simulink library "UserBlocks"  (R2014a)
settings: Solver=ode45  SolverMode=SingleTasking  StartTime=0.0  StopTime=10.0  RelTol=1e-3
values from neighbouring files (symbols this model uses):
  a = param.a    [DSC_Control_Analysis.m]    (also in DSC_Control_Analysis_Exp.m; DSC_Speed_Control_Analysis.m; EmpiricalTireCurves.m = 1.35; FFW_Fx.m = sqrt(curvature/(2*clothoidLength)))
  b = 1.15    [EmpiricalTireCurves.m]
  Cfls = Cfl    [EC_params_nissan.m]
  Crls = Crl    [EC_params_nissan.m]
  d0 = CSTR.d0    [Ext_MPCPara.m]
  freq = Fs/2*linspace(0,1,NFFT/2)    [AACplottingcode.m]    (also in If_alpha_tp_observer.m; If_alpha_tp_observer_for_c_code.m; If_alpha_tp_observer_shoreline.m)
  Iz = param.Iz    [DSC_Control_Analysis.m]    (also in DSC_Control_Analysis_Exp.m; DSC_Speed_Control_Analysis.m; EmpiricalTireCurves.m = 1300)
  K = 10    [EC_params_nissan.m]
  Ks = -10    [EC_params_nissan.m]
  Ksl = -10    [EC_params_nissan.m]
  Kt = 40000    [EC_params_nissan.m]
  Ku = -40000    [EC_params_nissan.m]
  m = 1724    [EmpiricalTireCurves.m]
  mu_s = mu_p    (= 0.6)    [EC_params_nissan.m]    (also in EmpiricalTireCurves.m = 0.55)
  Ns = 10    [EC_params_nissan.m]
  num = num+MTnum(m)    [Build_MtMuMy.m]
  q = 1    [EC_params_nissan.m]
  Taoh = CSTR.Taoh    [Ext_MPCPara.m]
  Ts = 0.002    [DSC_Control_Analysis.m]    (also in DSC_Control_Analysis_Exp.m; DSC_Speed_Control_Analysis.m; EC_params_nissan.m; Ext_MPCPara.m = SSD.Ts)
undefined symbols (not defined in the file or in its folder): acceAmp, ack, alphaFrontSteeringLimit, alphaFrontTable, bit, c, Cfl, Crl, CSTR, dden, deltaPsiDotGain, deltDist, den, denafilt, dnum, elaDotGain, filtera, filterb, frontAlphaLookup, frontForceLookup, FuelStartCalTime, FyFtable, gpsins, h, h_roll, hal_filter_den, hal_filter_num, hwx, hwy5, initAcce, initSpeed, isDriverNoise, lkparams, mapDataFull, mapMatchingParams, maxFrontForce, maxNumSegs, mdPtrs, numafilt, param, rearAlphaLookup, rfl, rfr, rrl, rrr, sglu, SIMP, simuCond, slimFxl, slimFxu, sliml, slimMll, slimMlr, slimMul, slimMur, slimu, sr, SSD, Standard, steering_limit ... (+7)
libraries: simulink x28, slrtlib x18, UserBlocks x6, slrtsoftinglib x6, MickLibBlocks x1, DriftControllerLibrary x1
(part 4 of 6)

== system UserBlocks/Sliding Surface Control Subsystem v1/Sliding Surface Controller function/getFyr ==
  B : Inport
  Vx : Inport  Port=2
  r : Inport  Port=3
  Gain1 : Gain  Gain=-b
  Product : Product  RndMeth=Zero
  Sum1 : Sum  Inputs=|++
  TireCurve : Lookup  InputValues=rearAlphaLookup
  Trigonometric Function : Trigonometry  Operator=atan2
  Fyr : Outport
  wires:
  TireCurve/1 -> Fyr/1
  B/1 -> Product/1
  r/1 -> Gain1/1
  Vx/1 -> Trigonometric Function/2, Product/2
  Sum1/1 -> Trigonometric Function/1
  Trigonometric Function/1 -> TireCurve/1
  Gain1/1 -> Sum1/2
  Product/1 -> Sum1/1

== system UserBlocks/Sliding Surface Control Subsystem v1/Sliding Surface Controller function/getSurface_S ==
  B : Inport
  r : Inport  Port=2
  Bnom : Inport  Port=3
  rnom : Inport  Port=4
  Gain : Gain  Gain=q
  Sum : Sum  Inputs=|+-
  Sum1 : Sum  Inputs=|+-
  Sum2 : Sum  Inputs=|-+
  Surface_S : Outport
  wires:
  Sum2/1 -> Surface_S/1
  Sum/1 -> Sum2/2
  Gain/1 -> Sum2/1
  Sum1/1 -> Gain/1
  Bnom/1 -> Sum1/2
  B/1 -> Sum1/1
  rnom/1 -> Sum/2
  r/1 -> Sum/1

== system UserBlocks/Sliding Surface Control Subsystem v1/Sliding Surface Controller function/get_d_control ==
  B : Inport
  Vx : Inport  Port=2
  r : Inport  Port=3
  alphaFcontrol : Inport  Port=4
  Gain : Gain  Gain=a
  Product1 : Product  RndMeth=Zero
  Sum : Sum  Inputs=|++
  Sum1 : Sum  Inputs=|+-
  Trigonometric Function : Trigonometry  Operator=atan2
  d_control : Outport
  wires:
  Sum1/1 -> d_control/1
  alphaFcontrol/1 -> Sum1/2
  Trigonometric Function/1 -> Sum1/1
  Vx/1 -> Trigonometric Function/2, Product1/2
  r/1 -> Gain/1
  B/1 -> Product1/1
  Sum/1 -> Trigonometric Function/1
  Gain/1 -> Sum/2
  Product1/1 -> Sum/1

== system UserBlocks/Steering Controller/HAL-9000/Chirp Signal ==
  note: freqSlope = deltaFreq/targetTime;
      | instantaneousFreq(t) = freqSlope*t + initialFreq;
      | intantaneousPhase(t) = integral(instFreq) = ...
      |       0.5*freqSlope*t^2 + initialFreq*t;
      | outputSignal(t) = sin(instantaneousPhase(t));
  Start Time : Inport
  Clock1 : Clock
      settings: DisableCoverage=on
  Gain : Gain  DisableCoverage=on  Gain=0.5  OutDataTypeStr=Inherit: Same as input  ParamDataTypeStr=Inherit: Same as input
  Output : Trigonometry
  Product : Product  DisableCoverage=on  Inputs=*/  SaturateOnIntegerOverflow=on  InputSameDT=on  OutDataTypeStr=Inherit: Same as first input
  Product1 : Product  DisableCoverage=on  SaturateOnIntegerOverflow=on  InputSameDT=on  OutDataTypeStr=Inherit: Same as first input
  Product2 : Product  DisableCoverage=on  SaturateOnIntegerOverflow=on  InputSameDT=on  OutDataTypeStr=Inherit: Same as first input
  Saturation : Saturate  UpperLimit=duration  LowerLimit=0
  Sum : Sum  DisableCoverage=on  Inputs=|++  SaturateOnIntegerOverflow=on  InputSameDT=on  OutDataTypeStr=Inherit: Same as first input
  Sum1 : Sum  DisableCoverage=on  Inputs=-+|  SaturateOnIntegerOverflow=on  InputSameDT=on  OutDataTypeStr=Inherit: Same as first input
  deltaFreq : Constant  DisableCoverage=on  Value=2*pi*(f2-f1)
  initialFreq : Constant  DisableCoverage=on  Value=2*pi*f1
  targetTime : Constant  DisableCoverage=on  Value=T
  Out2 : Outport
  wires:
  Saturation/1 -> Product2/1, Product1/1
  Output/1 -> Out2/1
  Product2/1 -> Output/1
  Sum/1 -> Product2/2
  initialFreq/1 -> Sum/2
  Product1/1 -> Sum/1
  Gain/1 -> Product1/2
  Product/1 -> Gain/1
  targetTime/1 -> Product/2
  deltaFreq/1 -> Product/1
  Start Time/1 -> Sum1/1
  Clock1/1 -> Sum1/2
  Sum1/1 -> Saturation/1

== system UserBlocks/Steering Controller/HAL-9000/Double chirp ==
  In1 : Inport
  Chirp One : Subsystem  mask(chirp){f1=startfreq, T=duration/2, f2=endfreq, VectorParams1D=on}
      mask prompts: f1 "Initial frequency (Hz):"; T "Target time (secs):"; f2 "Frequency at target time (Hz):"; VectorParams1D "Interpret vectors parameters as 1-D"
      mask help: Output a linear chirp signal (sine wave whose frequency varies linearly with time).
      mask init: same as UserBlocks/Steering Controller/HAL-9000/Chirp Signal
      mask Help: The chirp signal has linearly increasing frequency with time.  This block can be used for spectral analysis of nonlinear systems.
      mask Display: plot(t,sin(t.*t))
  Chirp Two : Subsystem  mask(chirp){f1=startfreq, T=duration/2, f2=endfreq, VectorParams1D=on}
      mask prompts: f1 "Initial frequency (Hz):"; T "Target time (secs):"; f2 "Frequency at target time (Hz):"; VectorParams1D "Interpret vectors parameters as 1-D"
      mask help: Output a linear chirp signal (sine wave whose frequency varies linearly with time).
      mask init: same as UserBlocks/Steering Controller/HAL-9000/Chirp Signal
      mask Help: The chirp signal has linearly increasing frequency with time.  This block can be used for spectral analysis of nonlinear systems.
      mask Display: plot(t,sin(t.*t))
  Clock : Clock
  Relational Operator : RelationalOperator  Operator=<=  OutDataTypeStr=float('double')
  Sum : Sum  DisableCoverage=on  Inputs=++|  SaturateOnIntegerOverflow=on  InputSameDT=on  OutDataTypeStr=Inherit: Same as first input
  Switch : Switch  Threshold=.5
  initialFreq : Constant  DisableCoverage=on  Value=duration/2
  Out1 : Outport
  wires:
  Chirp One/1(Out2) -> Switch/1
  Chirp Two/1(Out2) -> Switch/3
  Switch/1 -> Out1/1
  In1/1 -> Chirp One/1(Start Time), Sum/1
  Sum/1 -> Chirp Two/1(Start Time), Relational Operator/2
  initialFreq/1 -> Sum/2
  Relational Operator/1 -> Switch/2
  Clock/1 -> Relational Operator/1

== system UserBlocks/Steering Controller/HAL-9000/Double-step ==
  Start Time : Inport
  Clock : Clock
  Data Type Conversion : DataTypeConversion  OutDataTypeStr=double
  Data Type Conversion1 : DataTypeConversion  OutDataTypeStr=double
  Left Pulse : simulink/Logic and Bit Operations/Interval Test  IntervalClosedRight=off  uplimit=duration  IntervalClosedLeft=on  lowlimit=0  OutDataTypeStr=boolean
  Right Pulse : simulink/Logic and Bit Operations/Interval Test  IntervalClosedRight=off  uplimit=3*duration  IntervalClosedLeft=on  lowlimit=2*duration  OutDataTypeStr=boolean
  Sum : Sum  Inputs=+|-
  Sum1 : Sum  Inputs=+|-
  Out : Outport
  wires:
  Start Time/1 -> Sum/2
  Clock/1 -> Sum/1
  Sum/1 -> Left Pulse/1, Right Pulse/1
  Sum1/1 -> Out/1
  Right Pulse/1 -> Data Type Conversion1/1
  Left Pulse/1 -> Data Type Conversion/1
  Data Type Conversion/1 -> Sum1/1
  Data Type Conversion1/1 -> Sum1/2

== system UserBlocks/Steering Controller/HAL-9000/Latch ==
  In1 : Inport
  Trigger : TriggerPort
  Out1 : Outport
  wires:
  In1/1 -> Out1/1

== system UserBlocks/Steering Controller/HAL-9000/Ramp ==
  Start Time : Inport
  Clock : Clock
      settings: DisableCoverage=on
  Saturation : Saturate  UpperLimit=1  LowerLimit=0
  Slope : Gain  Gain=1/duration
  Sum : Sum  DisableCoverage=on  Inputs=|+-  SaturateOnIntegerOverflow=on  InputSameDT=on  OutDataTypeStr=Inherit: Same as first input
  Out1 : Outport
  wires:
  Clock/1 -> Sum/1
  Start Time/1 -> Sum/2
  Sum/1 -> Slope/1
  Saturation/1 -> Out1/1
  Slope/1 -> Saturation/1

== system UserBlocks/Steering Controller/HAL-9000/Step ==
  Start Time : Inport
  Clock : Clock
  Relational Operator : RelationalOperator  OutDataTypeStr=float('double')
  Out : Outport
  wires:
  Relational Operator/1 -> Out/1
  Clock/1 -> Relational Operator/1
  Start Time/1 -> Relational Operator/2

== system UserBlocks/TTS Steering Control/Compute Steering Along Path/FFWsteeringNonlinear ==
  SCACS : Inport
  States : Inport  Port=2
  axDesired : Inport  Port=3
  Bus Creator : BusCreator  Inputs=3
  Bus Selector1 : BusSelector  OutputSignals=Vx,axCG,Sideslip,Yaw Rate
  Bus Selector2 : BusSelector  OutputSignals=matchOut.crv,curOut.curSegType,curOut.curSegNum,curOut.curCrvI,curOut.curCrvF,curOut.curSegLngth
  Demux : Demux  Outputs=5
  Mux3 : Mux  Inputs=11
  S-Function : S-Function  FunctionName=FFWsteeringForceSS  Parameters=Cf,Cr,m,a,b,Iz,muPeak,muSlide,Ts, lam1, lam2, lam3, lam4  EnableBusSupport=off
  FFWfrontForce : Outport
  UySim : Outport  Port=2
  rSim : Outport  Port=3
  wires:
  Bus Selector2/6 -> Mux3/10  "<curSegLngth>"
  Bus Selector2/5 -> Mux3/9  "<curCrvF>"
  Bus Selector2/4 -> Mux3/8  "<curCrvI>"
  Demux/5 -> rSim/1  "rSim"
  Demux/4 -> UySim/1  "UySim"
  axDesired/1 -> Mux3/11
  Bus Selector2/3 -> Mux3/7  "<curSegNum>"
  Bus Selector2/2 -> Mux3/6  "<curSegType>"
  Mux3/1 -> S-Function/1
  Bus Selector2/1 -> Mux3/5  "<crv>"
  Bus Selector1/4 -> Mux3/4  "<Yaw Rate>"
  Bus Selector1/3 -> Mux3/3  "<Sideslip>"
  Bus Selector1/2 -> Mux3/2  "<axCG>"
  Bus Selector1/1 -> Mux3/1  "<Vx>"
  SCACS/1 -> Bus Selector2/1
  States/1 -> Bus Selector1/1
  S-Function/1 -> Demux/1
  Demux/1 -> Bus Creator/1  "FFW_Fyf"
  Demux/2 -> Bus Creator/2  "UyEstimate"
  Demux/3 -> Bus Creator/3  "rEstimate"
  Bus Creator/1 -> FFWfrontForce/1  "outputsFromFFWss"

== system UserBlocks/TTS Steering Control/Compute Steering Along Path/Feedback Steering Edit ==
  SCACS : Inport
  States : Inport  Port=2
  Abs : Abs
  Abs1 : Abs
  Bus Creator : BusCreator
  Bus Creator1 : BusCreator  Inputs=3
  Bus Creator2 : BusCreator  Inputs=3
  Bus Creator3 : BusCreator  Inputs=5
  Bus Creator4 : BusCreator  Inputs=2
  Bus Selector1 : BusSelector  OutputSignals=matchOut.e,matchOut.dPsi,matchOut.crv
  Bus Selector2 : BusSelector  OutputSignals=Vx,Sideslip,Yaw Rate
  Constant2 : Constant  Value=0  SampleTime=Ts
  Product : Product  RndMeth=Zero
  Product1 : Product  RndMeth=Zero
  Product2 : Product  Inputs=*/  RndMeth=Zero
  Sum : Sum  Inputs=-+|
  Sum2 : Sum  Inputs=++|
  Switch1 : Switch  Threshold=5
  Switch2 : Switch  Threshold=3*pi/180
  Terminator : Terminator
  a : Constant  Value=a
  calculate e_la : Fcn  Expr=( (a+u[3])*sin(u[2])+u[1] )*u[4]*cos(u[2])
  calculate ecopDot : Fcn  Expr=u[1]*cos(u[2])+u[3]*sin(u[2])+u[4]*u[5]
  calculate sDot : Fcn  Expr=u[2]*( cos(u[1])-tan(u[3])*sin(u[1]) )
  calculate vyCG : Fcn  Expr=u[1]*tan(u[2])
  convert to force : Gain  Gain=(param.fl.C+param.fr.C)  SaturateOnIntegerOverflow=on  OutDataTypeStr=Inherit: Same as input  ParamDataTypeStr=Inherit: Same as input
  delta psi dot gain : Gain  Gain=-1*deltaPsiDotGain  SampleTime=Ts  SaturateOnIntegerOverflow=on  OutDataTypeStr=Inherit: Same as input  ParamDataTypeStr=Inherit: Same as input
  e cop dot gain : Gain  Gain=-1*elaDotGain  SampleTime=Ts  SaturateOnIntegerOverflow=on  OutDataTypeStr=Inherit: Same as input  ParamDataTypeStr=Inherit: Same as input
  gain1 : Gain  Gain=lkparams.xla*.75  SaturateOnIntegerOverflow=on  OutDataTypeStr=Inherit: Same as input  ParamDataTypeStr=Inherit: Same as input
  pfk : Constant  Value=lkparams.pfk
  to make conversion consistent with the steering below : Gain  Gain=-2  SaturateOnIntegerOverflow=on  OutDataTypeStr=Inherit: Same as input  ParamDataTypeStr=Inherit: Same as input
  xla : Constant  Value=lkparams.xla
  xla1 : Constant  Value=3*pi/180
  xla3 : Constant  Value=lkparams.xla*.25
  deltaPsiDotFB : Outport
  steeringFBforce : Outport  Port=2
  wires:
  xla3/1 -> Sum2/1
  gain1/1 -> Sum2/2
  Product1/1 -> Terminator/1
  Abs/1 -> Product1/1
  Switch2/1 -> Bus Creator/3
  xla/1 -> Switch2/1
  e cop dot gain/1 -> Bus Creator2/3  "elaDotFBforce"
  calculate ecopDot/1 -> e cop dot gain/1
  a/1 -> Bus Creator3/4
  calculate vyCG/1 -> Bus Creator3/1
  Bus Creator4/1 -> calculate vyCG/1
  Bus Creator3/1 -> calculate ecopDot/1
  to make conversion consistent with the steering below/1 -> Bus Creator2/1  "LKsteeringFBforce"
  Bus Creator2/1 -> steeringFBforce/1  "steeringFBforce"
  convert to force/1 -> Bus Creator2/2  "deltaPsiDotFBforce"
  Bus Selector1/3 -> Product/1  "<crv>"
  States/1 -> Bus Selector2/1
  Bus Selector1/2 -> Switch2/2, Product1/2, Abs/1, Abs1/1, Bus Creator/2, Bus Creator3/2, Bus Creator1/1  "<dPsi>"
  Bus Selector1/1 -> Bus Creator/1  "<e>"
  calculate e_la/1 -> to make conversion consistent with the steering below/1
  pfk/1 -> Bus Creator/4
  Bus Creator/1 -> calculate e_la/1
  SCACS/1 -> Bus Selector1/1
  Bus Selector2/1 -> Bus Creator3/3, Bus Creator4/1, Switch1/2, Bus Creator1/2  "<Vx>"
  Bus Selector2/3 -> Sum/2  "<Yaw Rate>"
  Product/1 -> Sum/1
  Bus Selector2/2 -> Bus Creator4/2, Bus Creator1/3  "<Sideslip>"
  Bus Creator1/1 -> calculate sDot/1
  calculate sDot/1 -> Product/2
  Sum/1 -> Bus Creator3/5, delta psi dot gain/1  "deltaPsiDot"
  Constant2/1 -> Switch1/3
  delta psi dot gain/1 -> Switch1/1
  Switch1/1 -> convert to force/1, deltaPsiDotFB/1
  Abs1/1 -> Product2/1
  xla1/1 -> Product2/2
  Product2/1 -> gain1/1
  Sum2/1 -> Switch2/3

== system UserBlocks/TTS Steering Control/Compute Steering Along Path/Force2delta ==
  note: This Logic is used to prevent
      | vehicle from keep steering at the end
      | of the map
  note: only switch from simulation to estimate value
      | when the speed is above 2m/s
  note: if doing this way, without increasing mu
      | will not make alpha front go beyond alpha slide, what this
      | means is that it slip circle will never active laterally.
  FFWfrontBus : Inport
  FBsteeringForce : Inport  Port=2
  simValues : Inport  Port=3
  SCACS : Inport  Port=4
  States : Inport  Port=5
  Bus Creator : BusCreator  Inputs=3
  Bus Selector : BusSelector  OutputSignals=UySim,rSim
  Bus Selector1 : BusSelector  OutputSignals=LKsteeringFBforce,deltaPsiDotFBforce,elaDotFBforce
  Bus Selector2 : BusSelector  OutputSignals=FFW_Fyf,UyEstimate,rEstimate
  Bus Selector3 : BusSelector  OutputSignals=matchOut.dst2end
  Bus Selector4 : BusSelector  OutputSignals=Vx
  Constant : Constant  Value=0  SampleTime=Ts
  Constant1 : Constant  Value=0  SampleTime=Ts
  Gain : Gain  Gain=a
  Gain1 : Gain  Gain=a
  Product : Product  Inputs=*/  RndMeth=Zero
  Product2 : Product  Inputs=*/  RndMeth=Zero
  Relational Operator : RelationalOperator  Operator===  OutDataTypeStr=boolean  SampleTime=Ts
  Sum1 : Sum  Inputs=++++
  Sum2 : Sum
  Sum3 : Sum  Inputs=+-
  Sum4 : Sum
  Switch : Switch  Threshold=2
  Switch1 : Switch  Threshold=.5
  Trigonometric Function : Trigonometry  Operator=atan
  force2alphaFront : Lookup  InputValues=-FyFtable  Table=-alphaFrontTable  LookUpMeth=Interpolation-Use End Values
  deltaSteering : Outport
  FFWsteeringSSsignals : Outport  Port=2
  wires:
  Product/1 -> Switch/3
  Product2/1 -> Switch/1
  States/1 -> Bus Selector4/1
  Bus Selector/2 -> Gain1/1  "<rSim>"
  Bus Selector/1 -> Sum4/1  "<UySim>"
  simValues/1 -> Bus Selector/1
  SCACS/1 -> Bus Selector3/1
  Bus Selector3/1 -> Relational Operator/1  "<dst2end>"
  Constant/1 -> Relational Operator/2
  Relational Operator/1 -> Switch1/2
  Constant1/1 -> Switch1/1
  Switch1/1 -> deltaSteering/1
  Sum4/1 -> Product/1
  Sum2/1 -> Product2/1
  Switch/1 -> Trigonometric Function/1
  Gain1/1 -> Sum4/2
  Sum1/1 -> force2alphaFront/1
  FFWfrontBus/1 -> Bus Creator/2, Bus Selector2/1
  Bus Selector2/1 -> Sum1/1  "<FFW_Fyf>"
  Bus Selector2/2 -> Sum2/1  "<UyEstimate>"
  Bus Selector2/3 -> Gain/1  "<rEstimate>"
  FBsteeringForce/1 -> Bus Selector1/1, Bus Creator/3
  Bus Selector1/1 -> Sum1/2  "<LKsteeringFBforce>"
  Bus Selector1/2 -> Sum1/3  "<deltaPsiDotFBforce>"
  Bus Selector4/1 -> Product2/2, Switch/2, Product/2  "<Vx>"
  Gain/1 -> Sum2/2
  Trigonometric Function/1 -> Sum3/1
  force2alphaFront/1 -> Sum3/2  "alphaFront"
  Sum3/1 -> Switch1/3, Bus Creator/1  "deltaSS"
  Bus Creator/1 -> FFWsteeringSSsignals/1
  Bus Selector1/3 -> Sum1/4  "<elaDotFBforce>"

== system UserBlocks/TTS Steering Control/Compute Steering Along Path/Limited Steering ==
  States : Inport
  delta Command : Inport  Port=2
  Bus Creator : BusCreator  Inputs=5
  Bus Selector2 : BusSelector  OutputSignals=Sideslip,Yaw Rate,Vx
  Constant : Constant  Value=alphaFrontSteeringLimit  SampleTime=Ts
  S-Function3 : S-Function  FunctionName=limitSteering  Parameters=a  EnableBusSupport=off
  delta Command regulated : Outport
  wires:
  delta Command/1 -> Bus Creator/5
  Bus Selector2/3 -> Bus Creator/4  "<Vx>"
  Bus Selector2/2 -> Bus Creator/3  "<Yaw Rate>"
  Bus Selector2/1 -> Bus Creator/2  "<Sideslip>"
  Constant/1 -> Bus Creator/1
  S-Function3/1 -> delta Command regulated/1
  Bus Creator/1 -> S-Function3/1
  States/1 -> Bus Selector2/1

== system UserBlocks/TTS Steering Control/Compute Steering Along Path/StaticMap ==
  States : Inport
  Bus Creator : BusCreator  Inputs=20
  Constant1 : Constant  Value=mapDataFull
  MATLAB Function : MATLAB Function  TreatAsAtomicUnit=on
  Map-Matching Primatives Dynamic Map P1 : Subsystem
  map : Outport
  mapMatch : Outport  Port=2
  wires:
  MATLAB Function/2(segType) -> Bus Creator/2  "segType"
  MATLAB Function/16(fricUpdated) -> Bus Creator/16  "fricUpdated"
  MATLAB Function/15(fricBase) -> Bus Creator/15  "fricBase"
  MATLAB Function/14(maxV) -> Bus Creator/14  "maxV"
  MATLAB Function/13(maxE) -> Bus Creator/13
  MATLAB Function/12(bank) -> Bus Creator/12  "bank"
  MATLAB Function/11(grade) -> Bus Creator/11  "grade"
  MATLAB Function/10(kEnd) -> Bus Creator/10  "kEnd"
  MATLAB Function/9(kStart) -> Bus Creator/9  "kStart"
  MATLAB Function/8(psiInit) -> Bus Creator/8  "psiInit"
  MATLAB Function/7(Uinit) -> Bus Creator/7  "Uinit"
  MATLAB Function/6(Ninit) -> Bus Creator/6  "Ninit"
  MATLAB Function/5(Einit) -> Bus Creator/5  "Einit"
  MATLAB Function/4(cumLength) -> Bus Creator/4  "cumLength"
  MATLAB Function/3(segLength) -> Bus Creator/3  "segLength"
  MATLAB Function/1(segNum) -> Bus Creator/1  "segNum"
  Bus Creator/1 -> Map-Matching Primatives Dynamic Map P1/2(Map), map/1
  Constant1/1 -> MATLAB Function/1(mapData)
  MATLAB Function/17(segModType) -> Bus Creator/17
  MATLAB Function/18(mapType) -> Bus Creator/18  "mapType"
  MATLAB Function/19(totalLength) -> Bus Creator/19  "totalLength"
  MATLAB Function/20(totalSegs) -> Bus Creator/20  "totalSegs"
  Map-Matching Primatives Dynamic Map P1/1(Match Out) -> mapMatch/1
  States/1 -> Map-Matching Primatives Dynamic Map P1/1(States)

== system UserBlocks/TTS Steering Control/Compute Steering Along Path/desiredSpeed Dynamic Maps ==
  Map : Inport
  SCACS : Inport  Port=2
  Bus Selector1 : BusSelector  OutputSignals=totalSegs,mapType,segType,fricBase,bank,grade,kStart,kEnd,segLength
  Bus Selector3 : BusSelector  OutputSignals=curOut.curSegNum,curOut.curSegProg
  Demux : Demux  Outputs=2
  S-Function3 : S-Function  FunctionName=desiredUxAxDynamicMaps  Parameters=m,a,b,h,maxNumSegs  EnableBusSupport=off
  UxDesired : Outport
  AxDesired : Outport  Port=2
  wires:
  Bus Selector1/9 -> S-Function3/11  "<segLength>"
  Bus Selector1/8 -> S-Function3/10  "<kEnd>"
  Bus Selector1/7 -> S-Function3/9  "<kStart>"
  Bus Selector1/6 -> S-Function3/8  "<grade>"
  Bus Selector1/5 -> S-Function3/7  "<bank>"
  Bus Selector1/4 -> S-Function3/6  "<fricBase>"
  Bus Selector1/3 -> S-Function3/5  "<segType>"
  Bus Selector1/2 -> S-Function3/4  "<mapType>"
  Bus Selector1/1 -> S-Function3/3  "<totalSegs>"
  Bus Selector3/1 -> S-Function3/1  "<curSegNum>"
  SCACS/1 -> Bus Selector3/1
  S-Function3/1 -> Demux/1
  Demux/1 -> UxDesired/1
  Demux/2 -> AxDesired/1
  Bus Selector3/2 -> S-Function3/2  "<curSegProg>"
  Map/1 -> Bus Selector1/1

== system UserBlocks/Diagnostic System/Residual Generation/Controller Model/Ackermann Correction ==
  Ackermann Angle : Inport
  Mux : Mux  Inputs=2
  left ackermann ideal correction angle : Fcn  Expr=u/(1-u*ack*param.tw/2/(param.a+param.b))
  right ackermann ideal correction angle : Fcn  Expr=u/(1+u*ack*param.tw/2/(param.a+param.b))
  Steer Angles : Outport
  wires:
  Ackermann Angle/1 -> right ackermann ideal correction angle/1, left ackermann ideal correction angle/1
  right ackermann ideal correction angle/1 -> Mux/2
  Mux/1 -> Steer Angles/1
  left ackermann ideal correction angle/1 -> Mux/1

== system UserBlocks/Diagnostic System/Residual Generation/Controller Model/Steering Geometry & Gearbox Correction ==
  Steer Angles : Inport
  Demux : Demux  Outputs=2
  Left Steer Angle Look-up : Lookup  InputValues=sglu.fl.sa  SaturateOnIntegerOverflow=on
  Left Steering Ratio : Gain  Gain=param.fl.gr  SaturateOnIntegerOverflow=on  OutDataTypeStr=Inherit: Same as input  ParamDataTypeStr=Inherit: Same as input
  Mux4 : Mux  Inputs=2
  Right Steer Angle Look-up : Lookup  InputValues=sglu.fr.sa  SaturateOnIntegerOverflow=on
  Right Steering Ratio : Gain  Gain=param.fl.gr  SaturateOnIntegerOverflow=on  OutDataTypeStr=Inherit: Same as input  ParamDataTypeStr=Inherit: Same as input
  Shaft Angles : Outport
  wires:
  Steer Angles/1 -> Demux/1
  Demux/1 -> Left Steer Angle Look-up/1
  Demux/2 -> Right Steer Angle Look-up/1
  Left Steer Angle Look-up/1 -> Left Steering Ratio/1
  Right Steer Angle Look-up/1 -> Right Steering Ratio/1
  Left Steering Ratio/1 -> Mux4/1
  Right Steering Ratio/1 -> Mux4/2
  Mux4/1 -> Shaft Angles/1

== system UserBlocks/EnvEnv Connection/Compute delta Steer/MPC UDP Send/Logic ==
  note: Set prev_corrN to zero when initStep
  note: initStep when CL just turned on
  note: always initStep when CL is off
  prev_corrN : Inport
  enableCL : Inport  Port=2
  Abs : Abs
  Compare To Constant : simulink/Logic and Bit Operations/Compare To Constant  relop=<=  const=0.5  OutDataTypeStr=uint8  ZeroCross=off
  Compare To Constant1 : simulink/Logic and Bit Operations/Compare To Constant  relop=>  const=0.1  OutDataTypeStr=uint8  ZeroCross=off
  Constant : Constant
  Data Type Conversion : DataTypeConversion
  Detect Increase : simulink/Logic and Bit Operations/Detect Increase  vinit=0.0  InputProcessing=Inherited  OutDataTypeStr=uint8
  Logical Operator : Logic  Operator=OR  AllPortsSameDT=off  OutDataTypeStr=boolean
  Product1 : Product  RndMeth=Zero
  Sum : Sum  Inputs=+-|
  prev_corrN_OUT : Outport
  wires:
  Product1/1 -> prev_corrN_OUT/1
  prev_corrN/1 -> Product1/2
  Data Type Conversion/1 -> Sum/1
  Compare To Constant1/1 -> Product1/1
  Abs/1 -> Compare To Constant1/1
  Sum/1 -> Abs/1
  Constant/1 -> Sum/2
  Detect Increase/1 -> Logical Operator/2
  Compare To Constant/1 -> Logical Operator/1
  enableCL/1 -> Detect Increase/1, Compare To Constant/1
  Logical Operator/1 -> Data Type Conversion/1

== system UserBlocks/EnvEnv Connection/Compute delta Steer/MPC UDP Send/Start MPC Calculation ==
  SentData_IN : Inport
  Pack : slrtlib/UDP/Pack   datatypes={'double'}  byteAlign=1
  Send : slrtlib/UDP/Send   ipAddress=171.64.164.232  ipPort=25001  localPort=25001  vblLen=off  sampletime=-1
  SentData_OUT : Outport
  wires:
  Pack/1 -> Send/1
  SentData_IN/1 -> Pack/1, SentData_OUT/1

== system UserBlocks/Envelope control with Differential drive/envelope controller with DD/Tire force control/limit_cal ==
  muFz : Inport
  alpha : Inport  Port=2
  ExpSW : Inport  Port=3
  stabilize DD : Inport  Port=4
  Fx_limit_cal : Subsystem
  Fx_limit_cal1 : Subsystem
  MinMax{1..4} (4 alike) : MinMax  Inputs=2
  Mux1 : Mux
  Mux7 : Mux
  RL & RR max : Constant  Value=3
  RL & RR max1 : Constant  Value=3
  RL min : Constant  Value=0.75
  RL min1 : Constant  Value=0.75
  RR min : Constant  Value=0.75
  RR min1 : Constant  Value=0.75
  Selector1 : Selector  InputPortWidth=4  Indices=3
  Selector2 : Selector  InputPortWidth=4  Indices=3
  Selector3 : Selector  InputPortWidth=4
  Selector8 : Selector  InputPortWidth=4
  Sum : Sum  Inputs=|++
  Sum1 : Sum  Inputs=|++
  Switch1 : Switch  Threshold=0.5
  Switch4 : Switch  Threshold=0.5
  adjustGain : Gain  Gain=1/1100
  adjustGain1 : Gain  Gain=1/1100
  pedal offset : Constant  Value=1.75
  pedal offset1 : Constant  Value=1.75
  slip_limit_cal1 : Subsystem
  slim : Outport
  Txlim : Outport  Port=2
  Txlim drive : Outport  Port=3
  wires:
  slip_limit_cal1/2(slim drive) -> Fx_limit_cal1/2(slim drive)
  pedal offset1/1 -> Sum1/2
  adjustGain1/1 -> Sum1/1
  Sum1/1 -> Selector3/1, Selector2/1
  Mux1/1 -> Switch1/1
  RR min1/1 -> Mux1/4
  MinMax2/1 -> Mux1/3
  RL min1/1 -> Mux1/2
  MinMax3/1 -> Mux1/1
  RL & RR max1/1 -> MinMax3/2, MinMax2/2
  Selector2/1 -> MinMax2/1
  Selector3/1 -> MinMax3/1
  Fx_limit_cal1/1(Txlim drive) -> Fx_limit_cal/5(Txlim drive), Switch1/3, adjustGain1/1
  Switch1/1 -> Txlim drive/1
  stabilize DD/1 -> Fx_limit_cal/4(stabilize DD), slip_limit_cal1/2(stabilize DD)
  pedal offset/1 -> Sum/2
  adjustGain/1 -> Sum/1
  Sum/1 -> Selector1/1, Selector8/1
  Mux7/1 -> Switch4/1
  RR min/1 -> Mux7/4
  MinMax1/1 -> Mux7/3
  RL min/1 -> Mux7/2
  MinMax4/1 -> Mux7/1
  RL & RR max/1 -> MinMax1/2, MinMax4/2
  Selector1/1 -> MinMax1/1
  Selector8/1 -> MinMax4/1
  alpha/1 -> Fx_limit_cal1/1(alpha), Fx_limit_cal/1(alpha), slip_limit_cal1/1(alpha)
  muFz/1 -> Fx_limit_cal1/3(muFz), Fx_limit_cal/3(muFz), slip_limit_cal1/3(muFz)
  slip_limit_cal1/1(slim) -> slim/1, Fx_limit_cal/2(slim)
  ExpSW/1 -> Switch1/2, Switch4/2
  Fx_limit_cal/1(Txlim) -> adjustGain/1, Switch4/3
  Switch4/1 -> Txlim/1

== system UserBlocks/Envelope control with Differential drive/envelope controller with DD/Tire force control/s_cal  ==
  note: Vx
  Omega : Inport
  Vx : Inport  Port=2
  yaw rate : Inport  Port=3
  ExpSW : Inport  Port=4
  Add4 : Sum  Inputs=+-
  Add5 : Sum  Inputs=+-
  Butterworth Filter : DiscreteFilter  Numerator=filterb  Denominator=filtera  SampleTime=0.002
  Butterworth Filter1 : DiscreteFilter  Numerator=filterb  Denominator=filtera  SampleTime=0.002
  Demux4 : Demux
  Divide : Product  Inputs=*/
  Divide1 : Product  Inputs=*/
  Gain1 : Gain  Gain=rrl
  Gain2 : Gain  Gain=rrr
  Gain3 : Gain  Gain=c
  Manual Switch : ManualSwitch  CurrentSetting=0
  Manual Switch1 : ManualSwitch  CurrentSetting=0
  Mux : Mux  Inputs=2
  Product : Product  RndMeth=Zero
  Relational Operator : RelationalOperator  Operator=<  OutDataTypeStr=boolean
  Relational Operator1 : RelationalOperator  Operator=<  OutDataTypeStr=boolean
  Saturation : Saturate  UpperLimit=0.99  LowerLimit=-0.99
  Saturation1 : Saturate  UpperLimit=0.99  LowerLimit=-0.99
  Sum : Sum  Inputs=|+-
  Sum1 : Sum  Inputs=++|
  Switch : Switch  Threshold=0.5
  Switch1 : Switch  Threshold=0.5
  Terminator1 : Terminator
  Terminator2 : Terminator
  prevent zero : Subsystem
  prevent zero1 : Subsystem
  s : Outport
  wires:
  Butterworth Filter/1 -> Manual Switch1/2
  Butterworth Filter1/1 -> Manual Switch/2
  Manual Switch/1 -> Product/1
  Saturation1/1 -> Mux/1
  Saturation/1 -> Mux/2
  Relational Operator1/1 -> Switch1/2
  Switch1/1 -> prevent zero/1(In1)
  Relational Operator/1 -> Switch/2
  Switch/1 -> prevent zero1/1(In1)
  prevent zero1/1(Out1) -> Divide1/2
  prevent zero/1(Out1) -> Divide/2
  Vx/1 -> Manual Switch1/1, Butterworth Filter/1
  Demux4/3 -> Gain1/1
  Demux4/4 -> Gain2/1
  Add4/1 -> Divide/1
  Add5/1 -> Divide1/1
  Omega/1 -> Demux4/1
  Divide/1 -> Saturation1/1
  Divide1/1 -> Saturation/1
  Mux/1 -> s/1
  Demux4/1 -> Terminator2/1
  Demux4/2 -> Terminator1/1
  yaw rate/1 -> Manual Switch/1, Butterworth Filter1/1
  ExpSW/1 -> Product/2
  Product/1 -> Gain3/1
  Sum/1 -> Switch1/3, Add4/1, Relational Operator1/1
  Sum1/1 -> Switch/3, Add5/1, Relational Operator/1
  Gain3/1 -> Sum/2, Sum1/1
  Gain1/1 -> Switch1/1, Add4/2, Relational Operator1/2
  Gain2/1 -> Switch/1, Add5/2, Relational Operator/2
  Manual Switch1/1 -> Sum/1, Sum1/2

== system UserBlocks/Envelope control with Differential drive/envelope controller with DD/Tire force control/slip_limit ==
  s : Inport
  slim : Inport  Port=2
  Constant4 : Constant  Value=[0;0]
  Data Type Conversion : DataTypeConversion
  Data Type Conversion1 : DataTypeConversion
  Demux2 : Demux  Outputs=2
  Demux3 : Demux  Outputs=2
  Demux4 : Demux  Outputs=2
  Demux5 : Demux  Outputs=3
  Demux6 : Demux  Outputs=3
  Gain : Gain  Gain=[1 0 0 0;0 1 0 0;0 0 1 1;0 0 1 1]  Multiplication=Matrix(K*u)
  Manual Switch : ManualSwitch  CurrentSetting=0
  Mux1 : Mux  Inputs=5
  Mux2 : Mux  Inputs=5
  Mux3 : Mux  Inputs=2
  Mux8 : Mux  Inputs=3
  S-Function : S-Function  FunctionName=TECslipcont  Parameters=[Ksl, Kt]  EnableBusSupport=off
  S-Function1 : S-Function  FunctionName=TECslipcont  Parameters=[Ksl, Kt]  EnableBusSupport=off
  Selector1 : Selector  InputPortWidth=4  Indices=[2,1]
  Selector3 : Selector  InputPortWidth=4  Indices=[4 3]
  Selector4 : Selector  InputPortWidth=3  Indices=3
  Selector5 : Selector  InputPortWidth=3  Indices=3
  Switch2 : Switch  Threshold=0.5
  Terminator1 : Terminator
  Terminator2 : Terminator
  Unit Delay : UnitDelay  SampleTime=0.002
  Unit Delay1 : UnitDelay  SampleTime=0.002
  Zero-Order Hold : ZeroOrderHold  SampleTime=0.002
  Zero-Order Hold1 : ZeroOrderHold  SampleTime=0.002
  DebugTEC : Outport
  drive trq : Outport  Port=2
  wires:
  Switch2/1 -> drive trq/1
  Manual Switch/1 -> Switch2/3
  Gain/1 -> Manual Switch/1
  Mux8/1 -> Manual Switch/2, Gain/1, Switch2/1
  [TEC_sw] -> Switch2/2
  Selector3/1 -> Zero-Order Hold1/1
  Zero-Order Hold1/1 -> Demux4/1
  Zero-Order Hold/1 -> Demux3/1
  slim/1 -> Selector3/1, Selector1/1
  Demux2/2 -> Mux2/1
  Demux2/1 -> Mux1/1
  Selector1/1 -> Zero-Order Hold/1
  Constant4/1 -> Mux8/1
  s/1 -> Demux2/1
  Mux1/1 -> S-Function/1
  S-Function/1 -> Demux5/1, Selector4/1
  Demux5/2 -> Unit Delay/1
  Mux2/1 -> S-Function1/1
  S-Function1/1 -> Demux6/1, Selector5/1
  Demux6/2 -> Unit Delay1/1
  Demux5/1 -> Mux8/2
  Demux6/1 -> Mux8/3
  Demux3/1 -> Mux1/2
  Demux3/2 -> Mux1/3
  Demux4/1 -> Mux2/2
  Demux4/2 -> Mux2/3
  Demux5/3 -> Terminator2/1
  Demux6/3 -> Terminator1/1
  Mux3/1 -> DebugTEC/1
  Selector4/1 -> Mux3/1
  Selector5/1 -> Mux3/2
  Unit Delay/1 -> Mux1/5
  [sliplimit_sw] -> Data Type Conversion/1
  Unit Delay1/1 -> Mux2/5
  [sliplimit_sw] -> Data Type Conversion1/1
  Data Type Conversion/1 -> Mux1/4
  Data Type Conversion1/1 -> Mux2/4

== system UserBlocks/Envelope control with Differential drive/envelope controller with DD/Tire force control/steering control ==
  yaw rate : Inport
  beta : Inport  Port=2
  Vx : Inport  Port=3
  alphalimit : Inport  Port=4
  wheel angle : Inport  Port=5
  Demux1 : Demux  Outputs=2
  MinMax2 : MinMax
  MinMax3 : MinMax  Function=max
  Mux3 : Mux  Inputs=2
  Mux4 : Mux  Inputs=2
  Mux5 : Mux  Inputs=2
  Selector : Selector  InputPortWidth=2
  Zero-Order Hold4 : ZeroOrderHold  SampleTime=0.002
  delta limit cal : Subsystem
  wheel angle1 : Outport
  wires:
  Vx/1 -> delta limit cal/1(Vx)
  Zero-Order Hold4/1 -> Mux4/1
  MinMax3/1 -> wheel angle1/1
  Mux3/1 -> Demux1/1
  Demux1/2 -> Mux5/2
  Demux1/1 -> Mux4/2
  Mux5/1 -> MinMax3/1
  MinMax2/1 -> Mux5/1
  Mux4/1 -> MinMax2/1
  wheel angle/1 -> Zero-Order Hold4/1
  delta limit cal/2(lower lim) -> Mux3/2
  delta limit cal/1(upper lim) -> Mux3/1
  beta/1 -> delta limit cal/2(beta)
  yaw rate/1 -> delta limit cal/3(yaw rate)
  alphalimit/1 -> Selector/1
  Selector/1 -> delta limit cal/4(aflim)

== system UserBlocks/Envelope control with Differential drive/envelope controller with DD/Tire force control/torque limit ==
  "drive trq " : Inport
  Txlim : Inport  Port=2
  MinMax4 : MinMax  Inputs=2
  MinMax5 : MinMax  Function=max  Inputs=2
  MinMax6 : MinMax  Inputs=2
  MinMax7 : MinMax  Function=max  Inputs=2
  Mux1 : Mux  Inputs=3
  Selector1 : Selector  InputPortWidth=4  Indices=[1 2]
  Selector10 : Selector  InputPortWidth=4
  Selector11 : Selector  InputPortWidth=4  Indices=3
  Selector12 : Selector  InputPortWidth=4  Indices=2
  Selector13 : Selector  InputPortWidth=4  Indices=4
  Selector8 : Selector  InputPortWidth=4  Indices=3
  Selector9 : Selector  InputPortWidth=4  Indices=4
  drive trq : Outport
  wires:
  Selector1/1 -> Mux1/1
  Txlim/1 -> Selector11/1, Selector13/1, Selector12/1, Selector10/1
  "drive trq "/1 -> Selector1/1, Selector8/1, Selector9/1
  Mux1/1 -> drive trq/1
  MinMax7/1 -> Mux1/3
  MinMax5/1 -> Mux1/2
  Selector13/1 -> MinMax7/2
  MinMax6/1 -> MinMax7/1
  Selector11/1 -> MinMax6/2
  Selector9/1 -> MinMax6/1
  Selector12/1 -> MinMax5/2
  MinMax4/1 -> MinMax5/1
  Selector10/1 -> MinMax4/2
  Selector8/1 -> MinMax4/1

== system UserBlocks/Envelope control with Differential drive/envelope controller with DD/Tire state estimation/Load Transfer ==
  Fx : Inport
  Fy : Inport  Port=2
  Fz_fl : Fcn  Expr=(b*m*9.8-h_roll*u[1])*(tw_m/2*m*9.8-h_roll*u[2])/((a+b)*2*tw_m/2*m*9.8)
  Fz_fr : Fcn  Expr=(b*m*9.8-h_roll*u[1])*(tw_m/2*m*9.8+h_roll*u[2])/((a+b)*2*tw_m/2*m*9.8)
  Fz_rl : Fcn  Expr=(a*m*9.8+h_roll*u[1])*(tw_m/2*m*9.8-h_roll*u[2])/((a+b)*2*tw_m/2*m*9.8)
  Fz_rr : Fcn  Expr=(a*m*9.8+h_roll*u[1])*(tw_m/2*m*9.8+h_roll*u[2])/((a+b)*2*tw_m/2*m*9.8)
  Mux : Mux  Inputs=2
  Mux1 : Mux
  Fz : Outport
  wires:
  Fx/1 -> Mux/1
  Mux1/1 -> Fz/1
  Fz_rr/1 -> Mux1/4
  Fz_rl/1 -> Mux1/3
  Fz_fr/1 -> Mux1/2
  Fz_fl/1 -> Mux1/1
  Mux/1 -> Fz_fr/1, Fz_rl/1, Fz_rr/1, Fz_fl/1
  Fy/1 -> Mux/2

== system UserBlocks/Envelope control with Differential drive/envelope controller with DD/Tire state estimation/Tire slip angle ==
  delta : Inport
  beta : Inport  Port=2
  r : Inport  Port=3
  Vx : Inport  Port=4
  Add : Sum  Inputs=++-
  Add1 : Sum  Inputs=-+
  Constant : Constant  Value=a
  Constant1 : Constant  Value=b
  Divide : Product  Inputs=**/
  Divide1 : Product  Inputs=**/
  af : Outport
  ar : Outport  Port=2
  wires:
  Add1/1 -> ar/1
  Divide1/1 -> Add1/1
  Constant1/1 -> Divide1/1
  Add/1 -> af/1
  delta/1 -> Add/3
  Vx/1 -> Divide1/3, Divide/3
  beta/1 -> Add1/2, Add/2
  r/1 -> Divide1/2, Divide/2
  Divide/1 -> Add/1
  Constant/1 -> Divide/1

== system UserBlocks/Envelope control with Differential drive/envelope controller with DD/Tire state estimation/alpha_limit_cal ==
  muFz : Inport
  Gain : Gain  Gain=3/Cfls
  Gain1 : Gain  Gain=3/Crls
  MinMax : MinMax  Function=max
  MinMax1 : MinMax  Function=max
  Mux : Mux  Inputs=2
  Selector : Selector  InputPortWidth=4  Indices=[1:2]
  Selector1 : Selector  InputPortWidth=4  Indices=[3:4]
  Trigonometric Function : Trigonometry  Operator=atan
  Trigonometric Function1 : Trigonometry  Operator=atan
  alphalimit_hat : Outport
  wires:
  Mux/1 -> alphalimit_hat/1
  Trigonometric Function1/1 -> Mux/2
  Trigonometric Function/1 -> Mux/1
  Gain1/1 -> Trigonometric Function1/1
  MinMax1/1 -> Gain1/1
  Selector1/1 -> MinMax1/1
  Gain/1 -> Trigonometric Function/1
  MinMax/1 -> Gain/1
  Selector/1 -> MinMax/1
  muFz/1 -> Selector1/1, Selector/1

== system UserBlocks/Envelope control with Differential drive/envelope controller with DD/VSP_cal/prevent zero ==
  In1 : Inport
  Abs : Abs
  Constant : Constant  Value=1/3.6
  Product : Product  RndMeth=Zero
  Relational Operator : RelationalOperator  Operator=>  OutDataTypeStr=boolean
  Sign : Signum
  Switch : Switch  Threshold=0.5
  Switch1 : Switch  Threshold=0.5
  Unit Delay : UnitDelay  InitialCondition=1  SampleTime=Ts
  Out1 : Outport
  wires:
  Unit Delay/1 -> Switch1/3
  Switch1/1 -> Unit Delay/1, Product/2
  Product/1 -> Switch/3
  Sign/1 -> Switch1/1
  In1/1 -> Sign/1, Abs/1, Switch/1
  Abs/1 -> Relational Operator/1
  Constant/1 -> Product/1, Relational Operator/2
  Relational Operator/1 -> Switch1/2, Switch/2
  Switch/1 -> Out1/1

== system UserBlocks/Envelope control with Differential drive/envelope controller with DD/target making/driving_dynamics ==
  In1 : Inport
  Transfer Fcn2 : TransferFcn  Numerator=(2*pi*10)^2*[1 2*0.8*(2*pi*fomg) (2*pi*fomg)^2]  Denominator=(2*pi*fomg)^2*[1 2*0.8*(2*pi*10) (2*pi*10)^2]
  Out1 : Outport
  wires:
  Transfer Fcn2/1 -> Out1/1
  In1/1 -> Transfer Fcn2/1

== system UserBlocks/Envelope control with Differential drive/envelope controller with DD/target making/torque limit ==
  "drive trq " : Inport
  Txlim drive : Inport  Port=2
  MinMax4 : MinMax  Inputs=2
  MinMax5 : MinMax  Function=max  Inputs=2
  MinMax6 : MinMax  Inputs=2
  MinMax7 : MinMax  Function=max  Inputs=2
  Mux1 : Mux  Inputs=3
  Selector1 : Selector  InputPortWidth=4  Indices=[1 2]
  Selector10 : Selector  InputPortWidth=4
  Selector11 : Selector  InputPortWidth=4  Indices=3
  Selector12 : Selector  InputPortWidth=4  Indices=2
  Selector13 : Selector  InputPortWidth=4  Indices=4
  Selector8 : Selector  InputPortWidth=4  Indices=3
  Selector9 : Selector  InputPortWidth=4  Indices=4
  drive trq : Outport
  wires:
  Selector1/1 -> Mux1/1
  Txlim drive/1 -> Selector11/1, Selector13/1, Selector12/1, Selector10/1
  "drive trq "/1 -> Selector1/1, Selector8/1, Selector9/1
  Mux1/1 -> drive trq/1
  MinMax7/1 -> Mux1/3
  MinMax5/1 -> Mux1/2
  Selector13/1 -> MinMax7/2
  MinMax6/1 -> MinMax7/1
  Selector11/1 -> MinMax6/2
  Selector9/1 -> MinMax6/1
  Selector12/1 -> MinMax5/2
  MinMax4/1 -> MinMax5/1
  Selector10/1 -> MinMax4/2
  Selector8/1 -> MinMax4/1

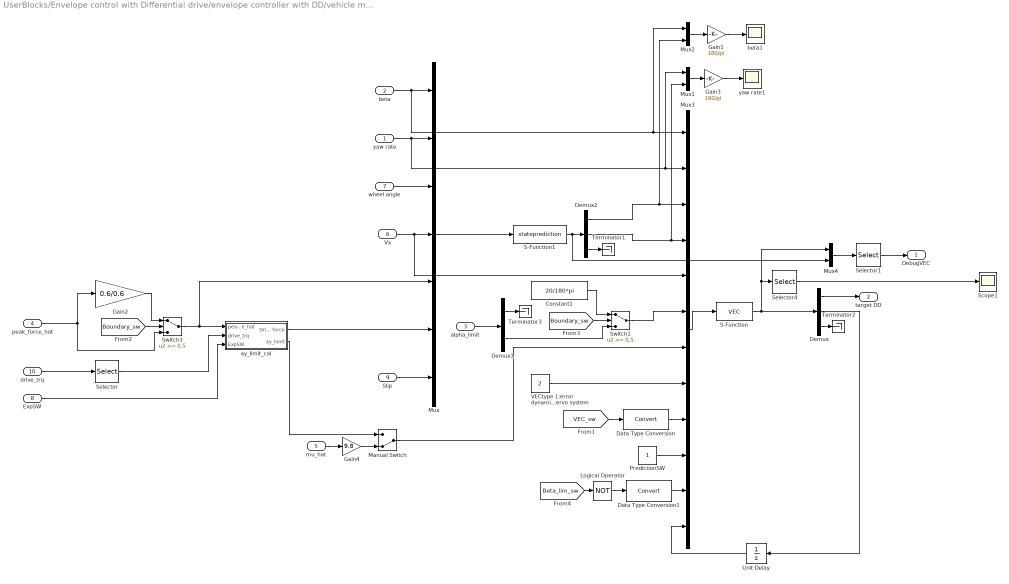
== system UserBlocks/Envelope control with Differential drive/envelope controller with DD/vehicle motion control/EC ==
  yaw rate : Inport
  beta : Inport  Port=2
  alpha_limit : Inport  Port=3
  peak_force_hat : Inport  Port=4
  mu_hat : Inport  Port=5
  Vx : Inport  Port=6
  wheel angle : Inport  Port=7
  ExpSW : Inport  Port=8
  Slip : Inport  Port=9
  drive_trq : Inport  Port=10
  Constant1 : Constant  Value=20/180*pi
  Data Type Conversion : DataTypeConversion
  Data Type Conversion1 : DataTypeConversion
  Demux : Demux  Outputs=[1 1 7]
  Demux1 : Demux  Outputs=2
  Demux2 : Demux  Outputs=3
  Gain1 : Gain  Gain=180/pi
  Gain2 : Gain  Gain=0.6/0.6
  Gain3 : Gain  Gain=180/pi
  Gain4 : Gain  Gain=9.8
  Logical Operator : Logic  Operator=NOT  AllPortsSameDT=off  OutDataTypeStr=boolean
  Manual Switch : ManualSwitch  CurrentSetting=0
  Mux : Mux  Inputs=7
  Mux1 : Mux  Inputs=2
  Mux2 : Mux  Inputs=2
  Mux3 : Mux  Inputs=12
  Mux4 : Mux  Inputs=2
  PredictionSW : Constant
  S-Function : S-Function  FunctionName=VEC  Parameters=[a,b,c,q,K,Ks,Ku]  EnableBusSupport=off
  S-Function1 : S-Function  FunctionName=stateprediction  Parameters=[a,b,c,Cfl,Crl,m,Iz]  EnableBusSupport=off
  Scope1 : Scope
      settings: TimeRange=20  YMin=0  YMax=25  SaveName=ScopeData3
  Selector : Selector  InputPortWidth=4  Indices=[3:4]
  Selector1 : Selector  InputPortWidth=12  Indices=[1:11]
  Selector4 : Selector  InputPortWidth=9  Indices=3
  Switch1 : Switch  Threshold=0.5
  Switch3 : Switch  Threshold=0.5
  Terminator1 : Terminator
  Terminator2 : Terminator
  Terminator3 : Terminator
  Unit Delay : UnitDelay  SampleTime=0.002
  VECtype 1:error dynamics 2:servo system : Constant  Value=2
  ay_limit_cal : Subsystem
  beta1 : Scope
      settings: YMin=-200  YMax=225  SaveName=ScopeData12
  yaw rate1 : Scope
      settings: TimeRange=20  YMin=0  YMax=25  SaveName=ScopeData10
  DebugVEC : Outport
  target DD : Outport  Port=2
  wires:
  Data Type Conversion1/1 -> Mux3/11
  Logical Operator/1 -> Data Type Conversion1/1
  [Beta_lim_sw] -> Logical Operator/1
  Unit Delay/1 -> Mux3/12
  Selector1/1 -> DebugVEC/1
  Mux4/1 -> Selector1/1
  PredictionSW/1 -> Mux3/10
  Data Type Conversion/1 -> Mux3/9
  VECtype 1:error dynamics 2:servo system/1 -> Mux3/8
  Manual Switch/1 -> Mux3/7
  Switch1/1 -> Mux3/6
  Demux2/2 -> Mux1/2, Mux3/4
  Demux2/1 -> Mux2/2, Mux3/3
  Slip/1 -> Mux/7
  ay_limit_cal/1(Driving force) -> Mux/6
  Vx/1 -> Mux3/5, Mux/4
  Demux1/1 -> Terminator3/1
  Demux2/3 -> Terminator1/1
  S-Function1/1 -> Mux4/2, Demux2/1
  Mux/1 -> S-Function1/1
  Mux3/1 -> S-Function/1
  Gain4/1 -> Manual Switch/2
  Selector4/1 -> Scope1/1
  Demux1/2 -> Switch1/3
  Constant1/1 -> Switch1/1
  [Boundary_sw] -> Switch1/2
  Gain2/1 -> Switch3/1
  Switch3/1 -> Mux/5, ay_limit_cal/1(peak_force_hat)
  [Boundary_sw] -> Switch3/2
  Mux2/1 -> Gain1/1
  Gain1/1 -> beta1/1
  Gain3/1 -> yaw rate1/1
  Mux1/1 -> Gain3/1
  mu_hat/1 -> Gain4/1
  ay_limit_cal/2(ay_limit) -> Manual Switch/1
  ExpSW/1 -> ay_limit_cal/3(ExpSW)
  alpha_limit/1 -> Demux1/1
  peak_force_hat/1 -> Switch3/3, Gain2/1
  Selector/1 -> ay_limit_cal/2(drive_trq)
  drive_trq/1 -> Selector/1
  yaw rate/1 -> Mux1/1, Mux3/2, Mux/2
  wheel angle/1 -> Mux/3
  Demux/1 -> target DD/1
  Demux/2 -> Unit Delay/1
  S-Function/1 -> Mux4/1, Selector4/1, Demux/1
  beta/1 -> Mux2/1, Mux3/1, Mux/1
  Demux/3 -> Terminator2/1
  [VEC_sw] -> Data Type Conversion/1

== system UserBlocks/LQACC/PIDACC/Car-Following System/Car-Follow Sys ==
  preSpd : Inport
  vehSpd : Inport  Port=2
  vehAcce : Inport  Port=3
  Des Dist : Subsystem
  I : Integrator  InitialConditionSource=external
  InitDist : Constant  Value=SIMP.x0(1)+Taoh*(Vpinit-SIMP.x0(2))+d0
  Step : Step  Time=stepTime  After=deltDist  SampleTime=0
  Sum : Sum  Inputs=|+-  SaturateOnIntegerOverflow=on
  Sum1 : Sum  Inputs=|+-  SaturateOnIntegerOverflow=on
  Sum2 : Sum  SaturateOnIntegerOverflow=on
  distErr : Outport
  relVel : Outport  Port=2
  vehACCE : Outport  Port=3
  dist : Outport  Port=4
  DesDist : Outport  Port=5
  wires:
  Sum1/1 -> I/1, relVel/1
  InitDist/1 -> I/2
  vehSpd/1 -> Des Dist/1(Vf), Sum1/2
  Des Dist/1(DesDist) -> Sum/2, DesDist/1
  vehAcce/1 -> vehACCE/1
  Sum/1 -> distErr/1
  preSpd/1 -> Sum1/1
  I/1 -> Sum2/2
  Sum2/1 -> Sum/1, dist/1
  Step/1 -> Sum2/1

== system UserBlocks/LQACC/PIDACC/MPC MTCACC/MTC ACC control ==
  PreAcce : Inport
  sysOuts : Inport  Port=2
  VehSpd : Inport  Port=3
  LQ controller1 : Subsystem
  Terminator : Terminator
  desAcce : Outport
  epsilon : Outport  Port=2
  wires:
  sysOuts/1 -> LQ controller1/2(sysOuts)
  PreAcce/1 -> LQ controller1/1(PreAcce)
  VehSpd/1 -> Terminator/1
  LQ controller1/1(desAccel) -> desAcce/1
  LQ controller1/2(epsilon) -> epsilon/1

== system UserBlocks/LQACC/PIDACC/PreVehicle/City Road StartTime=20s ==
  3.1 : Gain  Gain=-1  SaturateOnIntegerOverflow=on  OutDataTypeStr=Inherit: Same as input  ParamDataTypeStr=Inherit: Same as input
  3.2 : Gain  Gain=-1  SaturateOnIntegerOverflow=on  OutDataTypeStr=Inherit: Same as input  ParamDataTypeStr=Inherit: Same as input
  3.6 : Gain  Gain=-1  SaturateOnIntegerOverflow=on  OutDataTypeStr=Inherit: Same as input  ParamDataTypeStr=Inherit: Same as input
  Derivative : Derivative
  DirverNoise : Subsystem
  From Workspace2 : FromWorkspace  VariableName=[0,1;199.98,1;199.98,0;577.72,0]  SampleTime=0  Interpolate=off  OutputAfterFinalValue=Holding final value
  From Workspace5 : FromWorkspace  VariableName=[0,1;399.96,1;399.96,0;577.72,0]  SampleTime=0  Interpolate=off  OutputAfterFinalValue=Holding final value
  Integrator : Integrator
  Modification : Subsystem
  Saturation : Saturate  UpperLimit=30  LowerLimit=0
  Signal Generator : SignalGenerator  WaveForm=square  Amplitude=0.5  Frequency=1/33.33
  Signal Generator1 : SignalGenerator  WaveForm=square  Amplitude=0.5  Frequency=1/44.44
  Signal Generator2 : SignalGenerator  WaveForm=square  Amplitude=0.5  Frequency=1/22.22
  Switch : Switch  Threshold=0.5  SaturateOnIntegerOverflow=on
  Switch1 : Switch  Threshold=0.5  SaturateOnIntegerOverflow=on
  initSlope1 : Subsystem
  Alead : Outport
  Vlead : Outport  Port=2
  wires:
  DirverNoise/1(Out) -> Integrator/1
  Modification/1(Out) -> initSlope1/1(Xin)
  Integrator/1 -> Modification/1(in)
  initSlope1/1(Xout) -> Saturation/1
  From Workspace5/1 -> Switch1/2
  Signal Generator/1 -> 3.6/1
  From Workspace2/1 -> Switch/2
  Derivative/1 -> Alead/1
  Signal Generator2/1 -> 3.2/1
  Saturation/1 -> Derivative/1, Vlead/1
  Signal Generator1/1 -> 3.1/1
  3.6/1 -> Switch/1
  3.1/1 -> Switch1/3
  Switch1/1 -> Switch/3
  Switch/1 -> DirverNoise/1(In)
  3.2/1 -> Switch1/1

== system UserBlocks/LQACC/PIDACC/PreVehicle/Diff1 ==
  x : Inport
  RLimiter : RateLimiter  RisingSlewLimit=2  FallingSlewLimit=-2  SampleTimeMode=inherited
  TF2 : TransferFcn  Denominator=[0.3 1]
  d : Derivative
  dx : Outport
  wires:
  RLimiter/1 -> TF2/1
  TF2/1 -> dx/1
  d/1 -> RLimiter/1
  x/1 -> d/1

== system UserBlocks/LQACC/PIDACC/PreVehicle/Express Way StartTime=20s ==
  Constant2 : Constant  Value=0
  Derivative : Derivative
  DirverNoise : Subsystem
  From Workspace3 : FromWorkspace  VariableName=[0,0;435.06,0;437.12,1;611,1]  SampleTime=0  Interpolate=off  OutputAfterFinalValue=Holding final value
  From Workspace5 : FromWorkspace  VariableName=[0,1;220,1;220,0;1000,0]  SampleTime=0  Interpolate=off  OutputAfterFinalValue=Holding final value
  From Workspace6 : FromWorkspace  VariableName=[0,0;220,0;329,0;329,0.5;334.56,0.5;334.56,0;437.12,0;1000,0]  SampleTime=0  Interpolate=off  OutputAfterFinalValue=Holding final value
  From Workspace7 : FromWorkspace  VariableName=[611,0;711,0;711,-0.5;750,-0.5]  SampleTime=0  Interpolate=off  OutputAfterFinalValue=Holding final value
  From Workspace8 : FromWorkspace  VariableName=[0,1;611,1;611,0;1000,0]  SampleTime=0  Interpolate=off  OutputAfterFinalValue=Holding final value
  Integrator : Integrator
  Leading_vehicle : FromWorkspace  VariableName=[0,0; 5,0.5; 88.89,0;203.33,0;203.33,-0.5;220,-0.5]  SampleTime=0  OutputAfterFinalValue=Holding final value
  Modification : Subsystem
  Saturation : Saturate  UpperLimit=30  LowerLimit=0
  Signal Generator : SignalGenerator  WaveForm=square  Amplitude=0.4  Frequency=1/27.78
  Sum2 : Sum  Inputs=|++  SaturateOnIntegerOverflow=on
  Switch : Switch  Threshold=0.5  SaturateOnIntegerOverflow=on
  Switch1 : Switch  Threshold=0.5  SaturateOnIntegerOverflow=on
  Switch3 : Switch  Threshold=0.5  SaturateOnIntegerOverflow=on
  TFcn : TransferFcn  Denominator=[0.3 1]
  initSlope1 : Subsystem
  Alead : Outport
  Vlead : Outport  Port=2
  wires:
  DirverNoise/1(Out) -> Integrator/1
  initSlope1/1(Xout) -> Saturation/1
  Integrator/1 -> Modification/1(in)
  Modification/1(Out) -> initSlope1/1(Xin)
  Saturation/1 -> TFcn/1
  TFcn/1 -> Derivative/1, Vlead/1
  Derivative/1 -> Alead/1
  Switch3/1 -> Switch1/3
  From Workspace7/1 -> Switch3/3
  From Workspace8/1 -> Switch3/2
  Sum2/1 -> Switch3/1
  Switch/1 -> Sum2/1
  From Workspace6/1 -> Sum2/2
  Leading_vehicle/1 -> Switch1/1
  Constant2/1 -> Switch/3
  From Workspace5/1 -> Switch1/2
  Switch1/1 -> DirverNoise/1(In)
  Signal Generator/1 -> Switch/1
  From Workspace3/1 -> Switch/2

== system UserBlocks/LQACC/PIDACC/PreVehicle/initSlope ==
  Xin : Inport
  ConstVp : Constant  Value=Vpinit1
  ROperator : RelationalOperator  Operator=<=  OutDataTypeStr=boolean
  Ramp1 : simulink/Sources/Ramp  slope=initAcce  start=0  X0=initSpeed
  Switch3 : Switch  Threshold=0.5
  Xout : Outport
  wires:
  Switch3/1 -> Xout/1
  Xin/1 -> Switch3/1
  ROperator/1 -> Switch3/2
  Ramp1/1 -> Switch3/3, ROperator/2
  ConstVp/1 -> ROperator/1

== system UserBlocks/LQACC/PIDACC/PreVehicle/initSlope3 ==
  Xin : Inport
  ConstVp : Constant  Value=Vpinit5
  ROperator : RelationalOperator  Operator=<=  OutDataTypeStr=boolean
  Ramp1 : simulink/Sources/Ramp  slope=initAcce  start=0  X0=initSpeed
  Switch3 : Switch  Threshold=0.5
  Xout : Outport
  wires:
  ConstVp/1 -> ROperator/1
  Ramp1/1 -> ROperator/2, Switch3/3
  ROperator/1 -> Switch3/2
  Xin/1 -> Switch3/1
  Switch3/1 -> Xout/1

== system UserBlocks/LQACC/PIDACC/PreVehicle/sineAcce ==
  Product : Product  RndMeth=Zero
  Sine Pre Speed : Sin  Amplitude=acceAmp/(2*pi*freq)  Frequency=2*pi*freq  SampleTime=0
  Step : Step  Time=FuelStartCalTime  SampleTime=0
  Sum : Sum  Inputs=|++
  biasSpeed : Constant  Value=Vpinit5
  speed : Outport
  wires:
  Product/1 -> Sum/2
  biasSpeed/1 -> Sum/1
  Sum/1 -> speed/1
  Step/1 -> Product/2
  Sine Pre Speed/1 -> Product/1

== system UserBlocks/MPCACC/PIDACC/Car-Following System/Car-Follow Sys ==
  preSpd : Inport
  vehSpd : Inport  Port=2
  vehAcce : Inport  Port=3
  Des Dist : Subsystem
  I : Integrator  InitialConditionSource=external
  InitDist : Constant  Value=SIMP.x0(1)+Taoh*(Vpinit-SIMP.x0(2))+d0
  Step : Step  Time=stepTime  After=deltDist  SampleTime=0
  Sum : Sum  Inputs=|+-  SaturateOnIntegerOverflow=on
  Sum1 : Sum  Inputs=|+-  SaturateOnIntegerOverflow=on
  Sum2 : Sum  SaturateOnIntegerOverflow=on
  distErr : Outport
  relVel : Outport  Port=2
  vehACCE : Outport  Port=3
  dist : Outport  Port=4
  DesDist : Outport  Port=5
  wires:
  Step/1 -> Sum2/1
  Sum2/1 -> dist/1, Sum/1
  I/1 -> Sum2/2
  preSpd/1 -> Sum1/1
  Sum/1 -> distErr/1
  vehAcce/1 -> vehACCE/1
  Des Dist/1(DesDist) -> DesDist/1, Sum/2
  vehSpd/1 -> Sum1/2, Des Dist/1(Vf)
  InitDist/1 -> I/2
  Sum1/1 -> relVel/1, I/1
